simulink model "sampleModel1664"  (R2023a)
settings: Solver=VariableStepAuto  StartTime=0.0  StopTime=10.0  RelTol=1e-3
libraries: hdlsllib x6, simulink x4
settings Model: Creator=user1  LastModifiedBy=user1

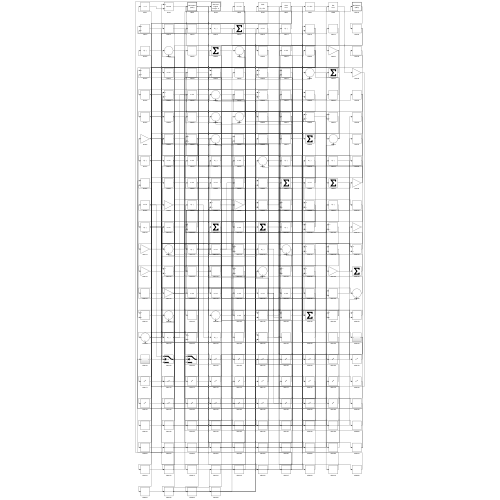
[thumbnail: Simulink's stored preview of the top-level diagram]
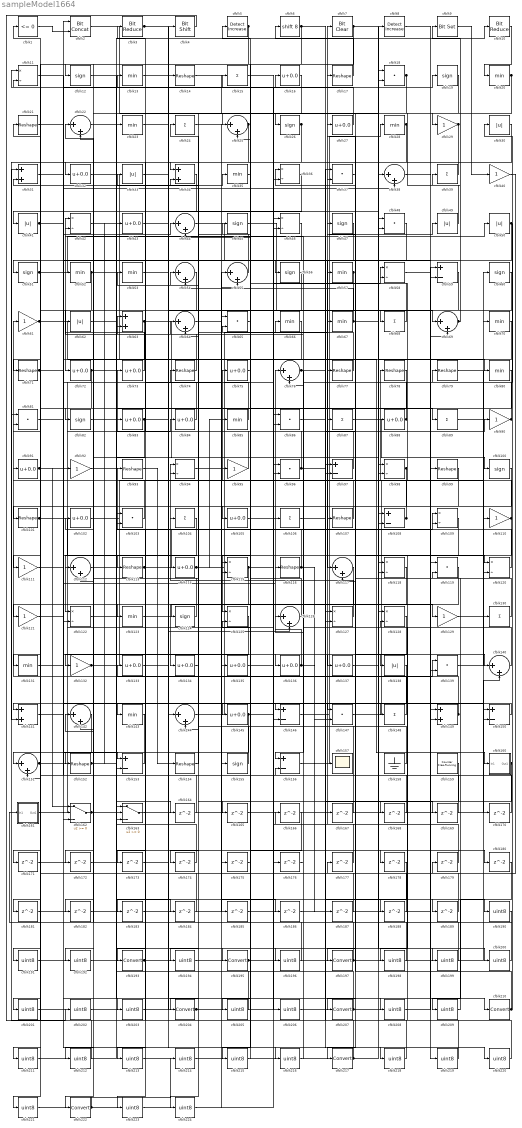
== system sampleModel1664 ==
  cfblk1 : hdlsllib/Logic and Bit Operations/Compare To Zero  relop=<=  OutDataTypeStr=boolean
  cfblk10 : hdlsllib/Logic and Bit Operations/Bit Reduce  mode=AND
  cfblk{12,19,26,45,47,51,56,60,82,100,124,155} (12 alike) : Signum
  cfblk{14,17,21,71,74,77..79,93,99,101,107,113,116,152,154} (16 alike) : Reshape
  cfblk{16,27,32,43,72..73,75,83..84,88,91,102,105,114,133..137,145} (20 alike) : Bias  Bias=0.0  SaturateOnIntegerOverflow=off
  cfblk{18,37,48,65,81,86,96,103,119,139,147} (11 alike) : DotProduct  OutDataTypeStr=Inherit: Inherit via internal rule
  cfblk{15,24,39,68,87,89,104,106,130,148} (10 alike) : Sum  Inputs=+
  cfblk{59,97,108,146,150,153,156} (7 alike) : Sum  Inputs=+-
  cfblk{11,36,42,46,58,94,98,109,115,118,120,122,125,127..128} (15 alike) : Product  Inputs=*/  RndMeth=Zero  SaturateOnIntegerOverflow=on
  cfblk{29,40,61,90,92,95,110..111,121,129,132} (11 alike) : Gain
  cfblk{22,25,38,44,54..55,64,69,76,112,117,126,140,142,144,151} (16 alike) : Sum  Inputs=|++
  cfblk{13,20,23,28,35,52..53,57,66..67,70,80,85,123,131,143} (16 alike) : MinMax
  cfblk{30,33,41,49..50,62,138} (7 alike) : Abs  SaturateOnIntegerOverflow=off
  cfblk{31,34,63,141,149} (5 alike) : Sum
  cfblk157 : Scope
  cfblk158 : Ground
  cfblk159 : hdlsllib/Sources/Counter Free-Running  NumBits=16  tsamp=-1
  cfblk160 : Subsystem
      settings: LibrarySourceBlock=|
      | hdlsllib/Ports &
      | Subsystems/Subsystem
  cfblk161 : Subsystem
      settings: LibrarySourceBlock=|
      | hdlsllib/Ports &
      | Subsystems/Subsystem
  cfblk162 : Switch  SaturateOnIntegerOverflow=off  InputSameDT=off
  cfblk163 : Switch  SaturateOnIntegerOverflow=off  InputSameDT=off
  cfblk{164..189} (26 alike) : Delay  SampleTime=1
  cfblk{190..192,194,196,198..203,205..206,208..209,211..216,218..221,223..224} (27 alike) : DataTypeConversion  OutDataTypeStr=uint8  SaturateOnIntegerOverflow=off  RndMeth=Floor
  cfblk{193,195,197,204,207,210,217,222} (8 alike) : DataTypeConversion  SaturateOnIntegerOverflow=off  RndMeth=Floor
  cfblk2 : hdlsllib/Logic and Bit Operations/Bit Concat  numInputs=2
  cfblk3 : hdlsllib/Logic and Bit Operations/Bit Reduce  mode=AND
  cfblk4 : hdlsllib/Logic and Bit Operations/Bit Shift  mode=Shift Left Logical  N=0
  cfblk5 : simulink/Logic and Bit Operations/Detect Increase  vinit=0.0  OutDataTypeStr=boolean
      settings: LibrarySourceBlock=|
      | hdlsllib/Logic and Bit
      | Operations/Detect
      | Increase
  cfblk6 : ArithShift  BitShiftNumber=8
  cfblk7 : simulink/Logic and Bit Operations/Bit Clear  iBit=0
      settings: LibrarySourceBlock=|
      | hdlsllib/Logic and Bit
      | Operations/Bit Clear
  cfblk8 : simulink/Logic and Bit Operations/Detect Increase  vinit=0.0  OutDataTypeStr=boolean
      settings: LibrarySourceBlock=|
      | hdlsllib/Logic and Bit
      | Operations/Detect
      | Increase
  cfblk9 : simulink/Logic and Bit Operations/Bit Set  iBit=0
      settings: LibrarySourceBlock=|
      | hdlsllib/Logic and Bit
      | Operations/Bit Set
  wires:
  cfblk99/1 -> cfblk193/1
  cfblk95/1 -> cfblk73/1
  cfblk93/1 -> cfblk154/1
  cfblk9/1 -> cfblk40/1
  cfblk32/1 -> cfblk160/1(In1)
  cfblk117/1 -> cfblk134/1
  cfblk7/1 -> cfblk12/1, cfblk115/1, cfblk199/1
  cfblk146/1 -> cfblk28/1
  cfblk148/1 -> cfblk61/1
  cfblk74/1 -> cfblk42/1
  cfblk151/1 -> cfblk83/1, cfblk116/1
  cfblk6/1 -> cfblk41/1, cfblk169/1
  cfblk85/1 -> cfblk63/1
  cfblk104/1 -> cfblk122/1
  cfblk136/1 -> cfblk76/1, cfblk147/2, cfblk187/1
  cfblk51/1 -> cfblk50/1, cfblk13/1
  cfblk49/1 -> cfblk25/1
  cfblk10/1 -> cfblk20/1
  cfblk29/1 -> cfblk141/1, cfblk97/2
  cfblk156/1 -> cfblk49/1
  cfblk54/1 -> cfblk72/1
  cfblk108/1 -> cfblk78/1, cfblk45/1
  cfblk77/1 -> cfblk53/1
  cfblk119/1 -> cfblk207/1
  cfblk152/1 -> cfblk43/1, cfblk164/1
  cfblk120/1 -> cfblk93/1
  cfblk127/1 -> cfblk94/1
  cfblk130/1 -> cfblk36/1
  cfblk162/1 -> cfblk139/1, cfblk184/1
  cfblk52/1 -> cfblk121/1, cfblk208/1
  cfblk76/1 -> cfblk156/1, cfblk168/1
  cfblk144/1 -> cfblk7/1
  cfblk110/1 -> cfblk58/1, cfblk117/2
  cfblk122/1 -> cfblk36/2
  cfblk140/1 -> cfblk42/2
  cfblk150/1 -> cfblk146/1
  cfblk115/1 -> cfblk180/1, cfblk201/1
  cfblk87/1 -> cfblk100/1
  cfblk70/1 -> cfblk112/1
  cfblk123/1 -> cfblk129/1
  cfblk50/1 -> cfblk79/1, cfblk144/2
  cfblk134/1 -> cfblk54/1
  cfblk103/1 -> cfblk22/1
  cfblk46/1 -> cfblk222/1
  cfblk1/1 -> cfblk2/2
  cfblk91/1 -> cfblk55/2, cfblk162/1
  cfblk79/1 -> cfblk130/1
  cfblk26/1 -> cfblk71/1, cfblk141/2
  cfblk111/1 -> cfblk44/1
  cfblk45/1 -> cfblk69/1
  cfblk163/1 -> cfblk17/1
  cfblk155/1 -> cfblk104/1
  cfblk56/1 -> cfblk82/1
  cfblk101/1 -> cfblk125/1, cfblk115/2, cfblk147/1
  cfblk69/1 -> cfblk39/1, cfblk9/1
  cfblk158/1 -> cfblk76/2
  cfblk18/1 -> cfblk107/1, cfblk182/1
  cfblk53/1 -> cfblk56/1
  cfblk139/1 -> cfblk60/1
  cfblk145/1 -> cfblk109/1, cfblk211/1
  cfblk27/1 -> cfblk11/2
  cfblk147/1 -> cfblk59/1
  cfblk38/1 -> cfblk140/1
  cfblk47/1 -> cfblk51/1
  cfblk41/1 -> cfblk59/2, cfblk120/2
  cfblk23/1 -> cfblk210/1
  cfblk113/1 -> cfblk8/1, cfblk139/2
  cfblk39/1 -> cfblk32/1
  cfblk13/1 -> cfblk14/1
  cfblk63/1 -> cfblk155/1, cfblk162/2
  cfblk36/1 -> cfblk111/1
  cfblk61/1 -> cfblk117/1, cfblk120/1
  cfblk149/1 -> cfblk114/1, cfblk148/1
  cfblk42/1 -> cfblk77/1
  cfblk21/1 -> cfblk16/1
  cfblk3/1 -> cfblk68/1, cfblk48/2
  cfblk116/1 -> cfblk5/1, cfblk157/1
  cfblk126/1 -> cfblk15/1
  cfblk67/1 -> cfblk54/2, cfblk80/1
  cfblk30/1 -> cfblk101/1
  cfblk48/1 -> cfblk127/2
  cfblk17/1 -> cfblk6/1
  cfblk84/1 -> cfblk33/1
  cfblk102/1 -> cfblk18/1
  cfblk22/1 -> cfblk98/2
  cfblk59/1 -> cfblk67/1
  cfblk33/1 -> cfblk144/1
  cfblk131/1 -> cfblk92/1
  cfblk90/1 -> cfblk47/1, cfblk63/2
  cfblk94/1 -> cfblk75/1
  cfblk98/1 -> cfblk151/1, cfblk122/2
  cfblk37/1 -> cfblk197/1
  cfblk14/1 -> cfblk26/1
  cfblk161/1(Out1) -> cfblk19/1
  cfblk121/1 -> cfblk74/1
  cfblk114/1 -> cfblk58/2, cfblk85/1
  cfblk55/1 -> cfblk31/2
  cfblk133/1 -> cfblk137/1
  cfblk124/1 -> cfblk102/1
  cfblk71/1 -> cfblk38/2, cfblk138/1
  cfblk107/1 -> cfblk91/1
  cfblk16/1 -> cfblk96/2
  cfblk154/1 -> cfblk24/1
  cfblk2/1 -> cfblk88/1
  cfblk132/1 -> cfblk70/1, cfblk84/1, cfblk109/2
  cfblk82/1 -> cfblk35/1
  cfblk28/1 -> cfblk113/1, cfblk108/2, cfblk57/1, cfblk162/3
  cfblk73/1 -> cfblk52/1
  cfblk159/1 -> cfblk204/1
  cfblk43/1 -> cfblk126/2
  cfblk19/1 -> cfblk29/1
  cfblk129/1 -> cfblk110/1
  cfblk83/1 -> cfblk192/1, cfblk196/1
  cfblk88/1 -> cfblk27/1, cfblk64/1
  cfblk81/1 -> cfblk136/1
  cfblk57/1 -> cfblk123/1, cfblk223/1
  cfblk112/1 -> cfblk10/1
  cfblk80/1 -> cfblk112/2
  cfblk11/1 -> cfblk153/1
  cfblk68/1 -> cfblk44/2
  cfblk62/1 -> cfblk195/1
  cfblk160/1(Out1) -> cfblk174/1, cfblk198/1
  cfblk153/1 -> cfblk152/1
  cfblk5/1 -> cfblk132/1, cfblk191/1
  cfblk65/1 -> cfblk105/1
  cfblk44/1 -> cfblk108/1
  cfblk92/1 -> cfblk163/3
  cfblk8/1 -> cfblk149/2
  cfblk25/1 -> cfblk131/1, cfblk64/2
  cfblk20/1 -> cfblk34/1, cfblk224/1
  cfblk128/1 -> cfblk217/1
  cfblk96/1 -> cfblk34/2, cfblk90/1
  cfblk34/1 -> cfblk143/1
  cfblk75/1 -> cfblk145/1
  cfblk125/1 -> cfblk142/2
  cfblk97/1 -> cfblk3/1
  cfblk15/1 -> cfblk150/2
  cfblk72/1 -> cfblk89/1, cfblk171/1
  cfblk164/1 -> cfblk11/1
  cfblk35/1 -> cfblk165/1
  cfblk165/1 -> cfblk150/1
  cfblk167/1 -> cfblk94/2
  cfblk168/1 -> cfblk1/1
  cfblk169/1 -> cfblk2/1
  cfblk89/1 -> cfblk170/1
  cfblk170/1 -> cfblk98/1
  cfblk171/1 -> cfblk153/2
  cfblk143/1 -> cfblk172/1
  cfblk172/1 -> cfblk142/1
  cfblk78/1 -> cfblk173/1
  cfblk174/1 -> cfblk163/2
  cfblk175/1 -> cfblk125/2
  cfblk176/1 -> cfblk156/2
  cfblk40/1 -> cfblk177/1
  cfblk177/1 -> cfblk126/1
  cfblk12/1 -> cfblk178/1
  cfblk179/1 -> cfblk96/1
  cfblk138/1 -> cfblk181/1
  cfblk181/1 -> cfblk163/1
  cfblk182/1 -> cfblk149/1
  cfblk60/1 -> cfblk183/1
  cfblk183/1 -> cfblk146/2
  cfblk184/1 -> cfblk81/2
  cfblk24/1 -> cfblk185/1
  cfblk185/1 -> cfblk25/2
  cfblk64/1 -> cfblk186/1
  cfblk186/1 -> cfblk127/1
  cfblk187/1 -> cfblk151/2
  cfblk109/1 -> cfblk188/1
  cfblk188/1 -> cfblk22/2
  cfblk137/1 -> cfblk189/1
  cfblk189/1 -> cfblk133/1
  cfblk86/1 -> cfblk190/1
  cfblk190/1 -> cfblk161/1(In1)
  cfblk191/1 -> cfblk86/1
  cfblk192/1 -> cfblk86/2
  cfblk193/1 -> cfblk176/1, cfblk175/1, cfblk38/1
  cfblk100/1 -> cfblk194/1
  cfblk194/1 -> cfblk99/1
  cfblk195/1 -> cfblk95/1, cfblk140/2
  cfblk196/1 -> cfblk62/1
  cfblk197/1 -> cfblk87/1, cfblk31/1
  cfblk198/1 -> cfblk37/1
  cfblk199/1 -> cfblk37/2
  cfblk135/1 -> cfblk200/1
  cfblk200/1 -> cfblk179/1
  cfblk201/1 -> cfblk135/1
  cfblk4/1 -> cfblk202/1
  cfblk202/1 -> cfblk124/1
  cfblk141/1 -> cfblk203/1
  cfblk203/1 -> cfblk4/1
  cfblk204/1 -> cfblk69/2, cfblk18/2
  cfblk166/1 -> cfblk205/1
  cfblk205/1 -> cfblk103/1
  cfblk105/1 -> cfblk206/1
  cfblk206/1 -> cfblk166/1
  cfblk207/1 -> cfblk48/1, cfblk65/1
  cfblk208/1 -> cfblk119/1
  cfblk180/1 -> cfblk209/1
  cfblk209/1 -> cfblk119/2
  cfblk210/1 -> cfblk167/1, cfblk30/1
  cfblk211/1 -> cfblk23/1
  cfblk118/1 -> cfblk212/1
  cfblk212/1 -> cfblk21/1
  cfblk178/1 -> cfblk213/1
  cfblk213/1 -> cfblk118/1
  cfblk214/1 -> cfblk118/2
  cfblk66/1 -> cfblk215/1
  cfblk215/1 -> cfblk65/2
  cfblk31/1 -> cfblk216/1
  cfblk216/1 -> cfblk66/1
  cfblk217/1 -> cfblk97/1, cfblk103/2
  cfblk173/1 -> cfblk218/1
  cfblk218/1 -> cfblk128/1
  cfblk58/1 -> cfblk219/1
  cfblk219/1 -> cfblk128/2
  cfblk106/1 -> cfblk220/1
  cfblk220/1 -> cfblk81/1
  cfblk142/1 -> cfblk221/1
  cfblk221/1 -> cfblk106/1
  cfblk222/1 -> cfblk214/1, cfblk55/1
  cfblk223/1 -> cfblk46/1
  cfblk224/1 -> cfblk46/2

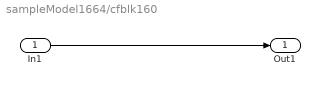
== system sampleModel1664/cfblk160 ==
  In1 : Inport
  Out1 : Outport
  wires:
  In1/1 -> Out1/1

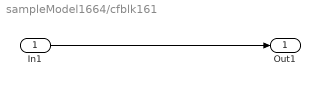
== system sampleModel1664/cfblk161 ==
  In1 : Inport
  Out1 : Outport
  wires:
  In1/1 -> Out1/1
